simulink model "doc_qpsk_rayleigh_derotated"  (R2014a)
settings: Solver=FixedStepDiscrete  StartTime=0.0  StopTime=inf  RelTol=1e-3
InitFcn:
  | seed_binary = 12345;
  | M=4;
  | EbNo=5;
  | randseed_AWGN = 12351;
  | seed_rayleigh = 12349;
  | maxNumErrs=1000;
  | maxNumBits=1e6;
undefined symbols (not defined in the file or in its folder): j
libraries: commchan3 x2, commdigbbndpm3 x2, commrandsrc2 x1, commsink2 x1
settings Model: Creator=The MathWorks Inc.
settings DataIOCC: SignalLoggingSaveFormat=ModelDataLogs
settings OptimizationCC: ExpressionDepthLimit=2147483647  InitFltsAndDblsToZero=on  EfficientMapNaN2IntZero=off
settings DebuggingCC: SaveWithParameterizedLinksMsg=none  UnderspecifiedInitializationDetection=Classic  SignalResolutionControl=TryResolveAllWithWarning  MultiTaskDSMMsg=warning  MultiTaskCondExecSysMsg=none  FcnCallInpInsideContextMsg=UseLocalSettings  StateNameClashWarn=warning  StrictBusMsg=None
settings RTWCC: IncludeERTFirstTime=on
settings GRTTargetCC: TargetFcnLib=ansi_tfl_tmw.mat  CombineOutputUpdateFcns=off  GRTInterface=on

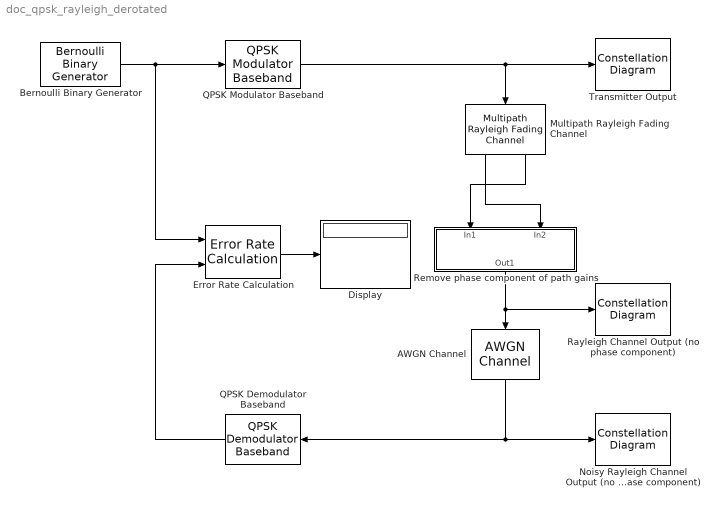
== system doc_qpsk_rayleigh_derotated ==
  AWGN Channel : commchan3/AWGN Channel  InputProcessing=Columns as channels (frame based)  seed=randseed_AWGN  noiseMode="Signal to noise ratio  (Eb/No)"  EbNodB=EbNo  EsNodB=10  SNRdB=EbNo+10*log10(log2(M))-10*log10((1e-6)/(1e-6))  bitsPerSym=log2(M)  Ps=1  Tsym=1e-6  variance=1
  Bernoulli Binary Generator : commrandsrc2/Bernoulli Binary Generator  P=0.5  seed=seed_binary  Ts=1e-6/log2(M)  frameBased=on  sampPerFrame=100*log2(M)  orient=off  outDataType=double
  Display : Display
  Error Rate Calculation : commsink2/Error Rate Calculation  N=0  st_delay=0  cp_mode=Entire frame  subframe=[]  PMode=Port  WsName=BER  RsMode2=off  stop=off  numErr=maxNumErrs  maxBits=maxNumBits
  Multipath Rayleigh Fading Channel : commchan3/Multipath Rayleigh Fading Channel  maxDopplerShift=1000  spectrumType=Jakes  sigmaGaussian=1/sqrt(2)  coeffRounded=[1 -1.72 0.785]  freqMinMaxRJakes=[0 1]  freqMinMaxAJakes=[0 1]  sigmaGaussian1=1/sqrt(2)  sigmaGaussian2=1/sqrt(2)  centerFreqGaussian1=0.0  centerFreqGaussian2=0.0  gainGaussian1=0.5  gainGaussian2=0.5  coeffBell=9  dopplerSpectrum=doppler.jakes  pathDelays=0  avgPathGaindB=0  normalizePathGains=on  seed=seed_rayleigh  enableProbe=0  openVisAtStart=off  outPathGains=on  outDelay=off
  Noisy Rayleigh Channel Output (no phase component) : ConstellationDiagram  Tag=ScatterPlot
  QPSK Demodulator Baseband : commdigbbndpm3/QPSK Demodulator Baseband  Ph=pi/4  Dec=Gray  OutType=Bit  DecType=Hard decision  VarSource=Dialog  Variance=1  outDtype1=double  outDtype2=double  derotateFactorWordLen=16
  QPSK Modulator Baseband : commdigbbndpm3/QPSK Modulator Baseband  InType=Bit  Enc=Gray  Ph=pi/4  outDtype=double  outWordLen=16  outUDDataType=sfix(16)  outFracLenMode=Best precision  outFracLen=15
  Rayleigh Channel Output (no phase component) : ConstellationDiagram  Tag=ScatterPlot
  Remove phase component of path gains : Subsystem
      mask Display: disp('Remove phase component\nof path gains')
  Transmitter Output : ConstellationDiagram  Tag=ScatterPlot
  wires:
  Bernoulli Binary Generator/1 -> Error Rate Calculation/1, QPSK Modulator Baseband/1
  QPSK Demodulator Baseband/1 -> Error Rate Calculation/2
  QPSK Modulator Baseband/1 -> Multipath Rayleigh Fading Channel/1, Transmitter Output/1
  Error Rate Calculation/1 -> Display/1
  AWGN Channel/1 -> Noisy Rayleigh Channel Output (no phase component)/1, QPSK Demodulator Baseband/1
  Multipath Rayleigh Fading Channel/2 -> Remove phase component of path gains/1(In1)
  Multipath Rayleigh Fading Channel/1 -> Remove phase component of path gains/2(In2)
  Remove phase component of path gains/1(Out1) -> AWGN Channel/1, Rayleigh Channel Output (no phase component)/1

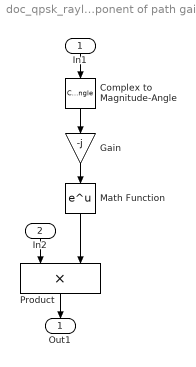
== system doc_qpsk_rayleigh_derotated/Remove phase component of path gains ==
  In1 : Inport
  In2 : Inport  Port=2
  Complex to Magnitude-Angle : ComplexToMagnitudeAngle  Output=Angle
  Gain : Gain  Gain=-j
  Math Function : Math  SaturateOnIntegerOverflow=on
  Product : Product  RndMeth=Zero
  Out1 : Outport
  wires:
  Complex to Magnitude-Angle/1 -> Gain/1
  Gain/1 -> Math Function/1
  Math Function/1 -> Product/2
  In1/1 -> Complex to Magnitude-Angle/1
  In2/1 -> Product/1
  Product/1 -> Out1/1
